simulink model "flightControlSystem"  (R2023a)
settings: Solver=ode3  StartTime=0  StopTime=TFinal  FixedStep=Ts  RelTol=1e-3  EnableMultiTasking=on
undefined symbols (not defined in the file): codertarget, Controller, DiscIntNeverNeededParam, Discrete, Estimator, g, gray, init, orient_ref, pos_ref, Rec, SDTV, Sensors, Time, Ts, var_acc_angle_N, var_bias_gyr_N, var_gyro_p_N, Vehicle
libraries: simulink x39, matrix_library x15, slpidlib x4, ctrlSharedLib x4, sharedtransform x3, visionconversions x2, visionfilter x1, parrotlib x1
(part 3 of 3)

== system flightControlSystem/Control System/State Estimator/XY Position Estimator/EstimatorVelocity/xy velocity w//o angular velocity compensation ==
  note: Optical flow raw readings are converted to velocity in m/s based on the estimated altitude
  optical_flow : Inport
  z_estimate : Inport  Port=2
  " " : Product  Inputs=**
  Compare To Constant : simulink/Logic and Bit Operations/Compare To Constant  relop=<  const=200*4  OutDataTypeStr=boolean
  Counter Free-Running : simulink/Sources/Counter Free-Running  NumBits=32  tsamp=-1
  Gain : Gain  Gain=-1
  Select dxy : Selector  InputPortWidth=3  IndexOptions=Index vector (dialog)  Indices=[1 2]  OutputSizes=1
  Switch : Switch  Criteria=u2 > Threshold  SaturateOnIntegerOverflow=off  InputSameDT=off
  opticalFlowErrorCorrect : Gain  Gain=1.15
  optical_flow_dx_dy : Outport
  wires:
  Select dxy/1 -> optical_flow_dx_dy/1  "optical_flow_dx_dy"
  " "/1 -> opticalFlowErrorCorrect/1
  opticalFlowErrorCorrect/1 -> Switch/3
  Gain/1 -> " "/2
  Switch/1 -> Select dxy/1
  Counter Free-Running/1 -> Compare To Constant/1
  Compare To Constant/1 -> Switch/2
  optical_flow/1 -> " "/1, Switch/1
  z_estimate/1 -> Gain/1

== matlab function flightControlSystem/Image Processing System/MATLAB Function ==
  data: Ii input; Io output; Io1 output; Ioo output
function [Io,Io1,Ioo]    = fcn(Ii)

Ii1 = imbinarize(Ii,'adaptive');

Ii2 = edge(Ii1,'canny');

se = strel('square',10);

Ii3 = imdilate(Ii2,se);

Ii4 = edge(Ii3,'canny');

Io = Ii4;
Io1 = Ii3;
Ioo = Ii4;

end

== matlab function flightControlSystem/Control System/Controller/Position Controller/Position error transformation (Earth to Body frame) ==
  data: yaw input; xy_err_earth input; xy_err_body output
function xy_err_body = fcn(yaw,xy_err_earth)

transformation = [cos(yaw), sin(yaw); -sin(yaw),  cos(yaw)];
xy_err_body = transformation * xy_err_earth;


end

== matlab function flightControlSystem/Image Processing System/MATLAB Function1 ==
  data: c input; theta_d output double; si input; ii input; sd input; id input; yaw input; a input; i input; d input; m output; thetaR output; im2 output; tot_mass output
function [theta_d,m,thetaR, im2,tot_mass] = fcn(c,si,ii,sd,id,yaw, a,i,d) %Estimar vel
    s1=sum(c,"all");
    s2=sum(si,"all");
    ii(:,20:31)=0;
    s3=sum(ii,"all");
    s4=sum(sd,"all");
    id(:,1:10)=0;
    s5=sum(id,"all");
    tot_mass=s1+s2+s3+s4+s5;
    c2=zeros(21,31);
    m=[si c sd;ii c2 id];

    sa=sum(a,"all");
    si=sum(i,"all");
    sd=sum(d,"all");
    c3=zeros(100,90);
    tot_mass2=sa+si+sd;
    
  
    mAux=[a;c3];
    im2=[i,mAux,d];
    
    [ii,jj] = ndgrid(1:size(im2,1),1:size(im2,2));
    R2 = sum(ii(:).*im2(:))/tot_mass2;
    C2 = sum(jj(:).*im2(:))/tot_mass2;

    %if tot_mass>20
        [ii,jj] = ndgrid(1:size(m,1),1:size(m,2));
        R = sum(ii(:).*m(:))/tot_mass;
        C = sum(jj(:).*m(:))/tot_mass;
        %Agregar un paso de 1 solo blob, probar con dif tamaños
        cr=41;%coord centrales dron
        cc=45;
        %x+
        m2=((R-cr)/(cc-C));
        %if R<cr
            if C>=cc
                ang=pi/2-atan(m2);
            else
                ang=-pi/2-atan(m2);
            end
        %{
        else
            if C>=cc
                ang=pi/2-atan(m2);
            else
                ang=-pi/2-atan(m2);
            end
        end
        %}
        %ang=pi/2-atan(m2); %coord normales desde cam
        thetaR=ang;
        theta=double(yaw)+ang;
    %{    
    theta=rem(theta,pi);
    thetaR=rem(thetaR,pi);
    
    if abs(theta)>pi
        theta=theta-sign(theta)*pi;
    end
    if abs(thetaR)>pi
        thetaR=thetaR-sign(thetaR)*pi;
    end
    %}
    %Logica vel
    %{
else
        %ExtraerBlobMasGrande
        R3=centroide(1);
        C3=centroide(2);
        cr=61;%coord centrales dron
        cc=80;
        %x+
        m2=((R3-cr)/(cc-C3));
        %if R<cr
        %{
            if C3>=cc
                ang=pi/2-atan(m2);
            else
                ang=-pi/2-atan(m2);
            end
        %}
        %{
        else
            if C>=cc
                ang=pi/2-atan(m2);
            else
                ang=-pi/2-atan(m2);
            end
        end
        %}
        %ang=pi/2-atan(m2); %coord normales desde cam
        
        %{
thetaR=ang;
        theta=yaw+ang;
        
        theta=rem(theta,pi);
        thetaR=rem(thetaR,pi);
        if abs(theta)>2.88
            theta=theta-sign(theta)*pi;
        end
        if abs(thetaR)>2.88
            thetaR=thetaR-sign(thetaR)*pi;
        end
        %}
        %}
    %end
theta_d=theta;

== matlab function flightControlSystem/Image Processing System/MATLAB Function3 ==
  data: li input; thetai output; si input; ld input; sd input; c input; thetad output; sumiC output; sumdC output; top output; m1 output; m2 output
function [thetai,thetad,sumiC,sumdC,top,m1,m2] = fcn(li,si,ld,sd,c)
m1=zeros(61,160);
m2=zeros(61,160);

m1(:,30:55)=li(1:61,30:end);
m1(1:20,36:85)=si;

m1C=zeros(120,160);
m1C(:,1:55)=li;
m1C(1:20,36:85)=si;
m1C(1:20,70:85)=0;

m2(:,106:131)=ld(1:61,1:26);
m2(1:20,75:125)=sd;

m2C=zeros(120,160);
m2C(:,106:end)=ld;
m2C(1:20,75:125)=sd;
m2C(1:20,75:90)=0;

sumdC=sum(m1C,"all");
sumiC=sum(m2C,"all");

sumi=sum(m1,"all");
sumd=sum(m2,"all");

top=sum(c,"all");


if(sumi>=20)
    [ii,jj] = ndgrid(1:size(m1,1),1:size(m1,2));
    Ri = sum(ii(:).*m1(:))/sumi;
    Ci = sum(jj(:).*m1(:))/sumi;
    
    cr=61;%coord centrales dron
    cc=80;
            %x+
    pend=((Ri-cr)/(cc-Ci));
    if Ci>=cc
        ang=pi/2-atan(pend);
    else
        ang=-pi/2-atan(pend);
    end
    thetai=ang;
else
    thetai=0;
end

if sumd>=20
    [ii,jj] = ndgrid(1:size(m2,1),1:size(m2,2));
    Rd = sum(ii(:).*m2(:))/sumd;
    Cd = sum(jj(:).*m2(:))/sumd;
    
    cr=61;%coord centrales dron
        cc=80;
    pend=((Rd-cr)/(cc-Cd));
        if Cd>=cc
            ang=pi/2-atan(pend);
        else
            ang=-pi/2-atan(pend);
        end
            thetad=ang;
else
    thetad=0;
end

== stateflow chart flightControlSystem/Control System/Path Planning/Chart ==
  state Logica de vuelo [group]
    state Despegue
      entry:
      x_pix = 0;
      y_pix = 0;
      z_com = -1.1;
      yaw_pix = 0;
      exit:
      z_com = -0.7;
    state status=posXd(x_pos) [function] [commented out]
      (default) -> (junction 711) [commented out]
      (junction 711) -> (junction 712) [commented out] : [x_pos >2.2]
      (junction 711) -> (junction 713) [commented out] : {status = 1;}
      (junction 712) -> (junction 714) [commented out] : {status = 0;}
      (junction 714) -> (junction 713) [commented out]
      (junction 713) -> (junction 715) [commented out]
    state Despegue1
      entry:
      x_pix = 0;
      y_pix = 0;
      z_com = -0.7;
      yaw_pix = 0;
      exit:
    state status = posXs(x_pos,x_d) [function] [commented out]
      (default) -> (junction 727) [commented out]
      (junction 727) -> (junction 728) [commented out] : [abs(x_pos-x_d)>0.01]
      (junction 727) -> (junction 729) [commented out] : {status = 0;}
      (junction 728) -> (junction 730) [commented out] : {status = 1;}
      (junction 730) -> (junction 729) [commented out]
      (junction 729) -> (junction 731) [commented out]
    state Avanzar4
      entry:
      yawd=yaw+(-1)*sign(yaw)*pi;%checar condiciones tengo que sumar, o invertir
      cy=yawd<yaw;
      ladoi=ci;
      ladod=cd;
      during:
      x_pix=0;
      y_pix=0;
      yaw_pix=-2*cy+1;
      thetaA=single(yawd);
      exit:
      x_pix = 0;
      yaw_pix=0;
      y_pix = 0;
    state status = rotYaw1(yaw) [function]
      (default) -> (junction 958)
      (junction 965) -> (junction 962) : [yaw>=yawd]
      (junction 958) -> (junction 966) [order 2] : [cy==1]
      (junction 958) -> (junction 965) [order 1] : [cy==0]
      (junction 966) -> (junction 953) : [yaw<=yawd]
      (junction 962) -> (junction 955) : {status=1;}
      (junction 953) -> (junction 952) : {status=1;}
      (junction 958) -> (junction 963) [order 3] : {status=0;}
      (junction 952) -> (junction 963)
      (junction 955) -> (junction 963)
      (junction 963) -> (junction 951)
    state Avanzar
      entry:
      dup=0;
      during:
      aux2=thetaR;%rem(thetaR,pi);
      x_pix=2.0*cos(double(theta_d));
      y_pix=2.0*sin(double(theta_d));
      dup=0;
      if s1>s2 && s1>150
      dup=1;
      ci=true;
      cd=false;
      else
      if s2>150
      dup=1;
      ci=false;
      cd=true;
      end
      end
      yaw_pix=aux2;
      thetaA=single(thetaR);
      exit:
      x_pix = 0;
      yaw_pix=0;
      y_pix = 0;
    state Avanzar5
      entry:
      during:
      aux2=thetaR;%rem(thetaR,pi);
      x_pix=1.5*cos(double(theta_d));
      y_pix=1.5*sin(double(theta_d));
      yaw_pix=aux2;
      thetaA=single(thetaR);
      exit:
      x_pix = 0;
      yaw_pix=0;
      y_pix = 0;
    state status = rotYaw(yaw,theta_d) [function] [commented out]
      (default) -> (junction 743) [commented out]
      (junction 743) -> (junction 744) [commented out] : [abs(yaw-theta_d) >= 0.1]
      (junction 743) -> (junction 745) [commented out] : {status = 0;}
      (junction 744) -> (junction 746) [commented out] : {status = 1;}
      (junction 746) -> (junction 745) [commented out]
      (junction 745) -> (junction 747) [commented out]
    state Avanzar6
      entry: %simC 30 funciona
      during:
      aux=thetai;%double(rem(thetai,pi));
      x_pix=1.5*cos(double(yaw+thetai));
      y_pix=1.5*sin(double(yaw+thetai));
      yaw_pix=aux;
      thetaA=single(thetai);
      exit:
      x_pix = 0;
      yaw_pix=0;
      y_pix = 0;
    state Avanzar7
      entry:
      during:
      aux=thetad;%double(rem(thetad,pi));
      x_pix=1.5*cos(double(yaw+thetad));
      y_pix=1.5*sin(double(yaw+thetad));
      yaw_pix=aux;
      thetaA=single(thetad);
      exit:
      x_pix = 0;
      yaw_pix=0;
      y_pix = 0;
    state status = posXd2(z_pos) [function] [commented out]
      (default) -> (junction 758) [commented out]
      (junction 758) -> (junction 759) [commented out] : [z_pos < -0.3]
      (junction 758) -> (junction 760) [commented out] : {status = 0;}
      (junction 759) -> (junction 761) [commented out] : {status = 1;}
      (junction 761) -> (junction 760) [commented out]
      (junction 760) -> (junction 762) [commented out]
    state Avanzar3
      during:
      x_pix = 0;
      y_pix = 0;
      z_com = -0.3;
      exit:
      x_pix = 0;
      y_pix = 0;
    state status = posXs2(y_pos,y_d) [function] [commented out]
      (default) -> (junction 774) [commented out]
      (junction 774) -> (junction 775) [commented out] : [abs(y_pos-y_d)> 0.01]
      (junction 774) -> (junction 776) [commented out] : {status = 0;}
      (junction 775) -> (junction 777) [commented out] : {status = 1;}
      (junction 777) -> (junction 776) [commented out]
      (junction 776) -> (junction 778) [commented out]
    state Aterriza
      during:
      x_pix = 0;
      y_pix = 0;
      z_com = 0;
      exit:
      x_pix = 0;
      y_pix = 0;
    (default) -> Despegue
    Despegue -> Despegue1 : [abs(abs(z_pos)-1.1)<0.05]
    Despegue1 -> Avanzar : [abs(abs(z_pos)-0.7)<0.01]
    Avanzar -> Avanzar4 [order 2] : [tot_mass<500]
    Avanzar7 -> Avanzar4 [order 1] : [tot_mass<500]
    Avanzar6 -> Avanzar4 [order 1] : [tot_mass<500]
    Avanzar4 -> (junction 995) : [rotYaw1(yaw)]
    Avanzar6 -> Avanzar [order 2] : [sumiC<=50]
    (junction 995) -> Avanzar5 : [after(2,sec)]
    Avanzar -> Avanzar7 [order 3] : [dup&&ci&&thetad~=0]
    Avanzar7 -> Avanzar [order 2] : [sumdC<=50]
    Avanzar -> Avanzar6 [order 4] : [dup&&cd&&thetai~=0]
    Avanzar -> Avanzar3 [order 1] : [F]
    Avanzar5 -> (junction 972) : [c<30]
    (junction 972) -> Avanzar6 [order 1] : [ladod]
    (junction 972) -> Avanzar7 [order 2] : [ladoi]
    Avanzar3 -> Aterriza : after(3,sec)[z_pos>-0.3]
  data: x_pos function_input; status function_output; x_pos function_input; status function_output; x_d function_input; yaw function_input; status function_output; yaw function_input; status function_output; theta_d function_input; z_pos function_input; status function_output; y_pos function_input; status function_output; y_d function_input; x_pix output; y_pix output; yaw_pix output; z_com output; z_pos input; theta_d input; F input; thetaA output; thetaR input; aux local; yaw input; yawd local; c input; thetad input; thetai input; tot_mass input; ladod local; ladoi local; aux2 local; s1 input; s2 input; ci data_store_memory; cd data_store_memory; dup local; cy local; sumdC input; sumiC input

== matlab function flightControlSystem/Image Processing System/MATLAB Function4 ==
  data: m1 input; s1 output; m2 input; s2 output; m output
function [s1,s2,m]= fcn(m1,m2)
s1=sum(m1,"all");
s2=sum(m2,"all");


c2=zeros(60,90);
m=[m1 c2 m2];
